simulink model "SEIRv2"  (R2019b)
settings: Solver=VariableStepAuto  StartTime=0.0  StopTime=365  FixedStep=1/24  RelTol=1e-6
settings Model: Creator=Alex  LastModifiedBy=Alex

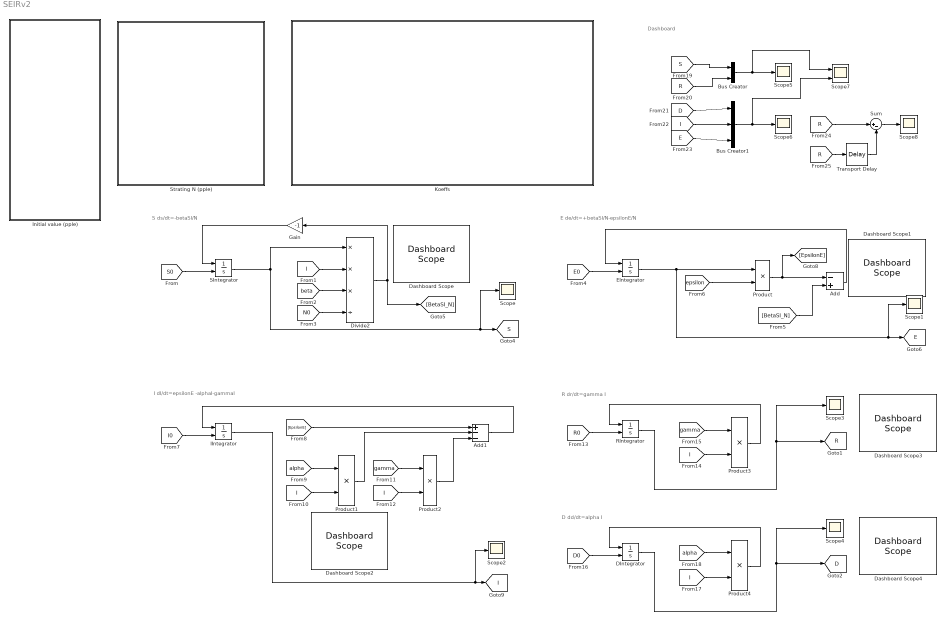
== system SEIRv2 ==
  note: Dashboard
  note: R dr/dt=gamma I
  note: I dI/dt=epsilonE -alphaI-gammaI
  note: E de/dt=+betaSI/N-epsilonE/N
  note: S ds/dt=-betaSI/N
  note: D dd/dt=alpha I
  Add : Sum  Inputs=-+
  Add1 : Sum  Inputs=+--
  Bus Creator : BusCreator  Inputs=2
  Bus Creator1 : BusCreator  Inputs=3
  DIntegrator : Integrator  InitialConditionSource=external
  Dashboard Scope{,1..4} (5 alike) : DashboardScope  Ymax=150e6
  Divide2 : Product  Inputs=***/
  EIntegrator : Integrator  InitialConditionSource=external
  Gain : Gain  Gain=-1
  IIntegrator : Integrator  InitialConditionSource=external
  Initial value (pple) : Subsystem
  Koeffs : Subsystem
  Product{,1..4} (5 alike) : Product  Inputs=**
  RIntegrator : Integrator  InitialConditionSource=external
  SIntegrator : Integrator  InitialConditionSource=external
  Scope{,1..6,8} (8 alike) : Scope
  Scope7 : Scope  NumInputPorts=2
  Strating N (pple) : Subsystem
  Sum : Sum  Inputs=|+-
  Transport Delay : TransportDelay
  tag scope: D=global, E=global, I=global, R=global, S=global
  wires:
  [S0] -> SIntegrator/2
  SIntegrator/1 -> Scope/1, [S], Divide2/1
  [I] -> Divide2/2
  [beta] -> Divide2/3
  [N0] -> Divide2/4
  Divide2/1 -> [BetaSI_N], Gain/1
  Gain/1 -> SIntegrator/1
  [E0] -> EIntegrator/2
  EIntegrator/1 -> Scope1/1, [E], Product/1
  [epsilon] -> Product/2
  Product/1 -> [EpsilonE], Add/1
  [BetaSI_N] -> Add/2
  Add/1 -> EIntegrator/1
  [I0] -> IIntegrator/2
  IIntegrator/1 -> [I], Scope2/1
  [alpha] -> Product1/1
  [I] -> Product1/2
  [gamma] -> Product2/1
  [I] -> Product2/2
  Product2/1 -> Add1/3
  Product1/1 -> Add1/2
  [EpsilonE] -> Add1/1
  Add1/1 -> IIntegrator/1
  [R0] -> RIntegrator/2
  RIntegrator/1 -> Scope3/1, [R]
  [gamma] -> Product3/1
  [I] -> Product3/2
  Product3/1 -> RIntegrator/1
  Product4/1 -> DIntegrator/1
  [I] -> Product4/2
  [alpha] -> Product4/1
  DIntegrator/1 -> [D], Scope4/1
  [D0] -> DIntegrator/2
  [S] -> Bus Creator/1
  [R] -> Bus Creator/2
  [D] -> Bus Creator1/1
  [I] -> Bus Creator1/2
  [E] -> Bus Creator1/3
  Bus Creator/1 -> Scope7/1, Scope5/1
  Bus Creator1/1 -> Scope7/2, Scope6/1
  [R] -> Transport Delay/1
  [R] -> Sum/1
  Transport Delay/1 -> Sum/2
  Sum/1 -> Scope8/1

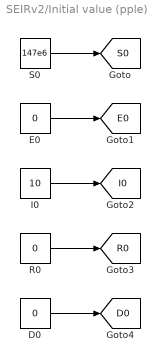
== system SEIRv2/Initial value (pple) ==
  D0 : Constant  Value=0
  E0 : Constant  Value=0
  I0 : Constant  Value=10
  R0 : Constant  Value=0
  S0 : Constant  Value=147e6
  tag scope: D0=global, E0=global, I0=global, R0=global, S0=global
  wires:
  S0/1 -> [S0]
  I0/1 -> [I0]
  D0/1 -> [D0]
  E0/1 -> [E0]
  R0/1 -> [R0]

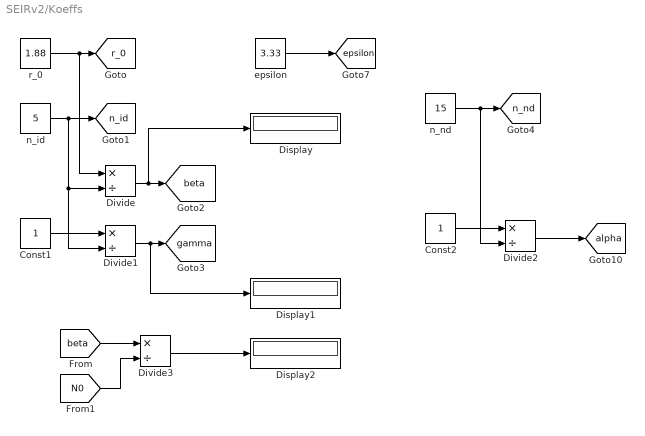
== system SEIRv2/Koeffs ==
  Const1 : Constant
  Const2 : Constant
  Display : Display
  Display1 : Display
  Display2 : Display
  Divide{,1..3} (4 alike) : Product  Inputs=*/
  epsilon : Constant  Value=3.33
  n_id : Constant  Value=5
  n_nd : Constant  Value=15
  r_0 : Constant  Value=1.88
  tag scope: alpha=global, beta=global, epsilon=global, gamma=global, n_id=global, n_nd=global, r_0=global
  wires:
  r_0/1 -> Divide/1, [r_0]
  Divide1/1 -> Display1/1, [gamma]
  n_id/1 -> Divide1/2, Divide/2, [n_id]
  Divide/1 -> Display/1, [beta]
  Const1/1 -> Divide1/1
  epsilon/1 -> [epsilon]
  Const2/1 -> Divide2/1
  Divide2/1 -> [alpha]
  n_nd/1 -> [n_nd], Divide2/2
  [beta] -> Divide3/1
  [N0] -> Divide3/2
  Divide3/1 -> Display2/1

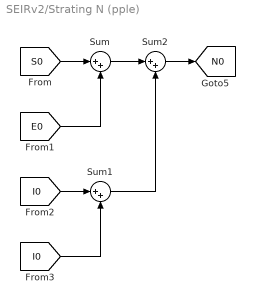
== system SEIRv2/Strating N (pple) ==
  Sum : Sum  Inputs=|++
  Sum1 : Sum  Inputs=|++
  Sum2 : Sum  Inputs=|++
  tag scope: N0=global
  wires:
  [I0] -> Sum1/1
  [S0] -> Sum/1
  [E0] -> Sum/2
  [I0] -> Sum1/2
  Sum2/1 -> [N0]
  Sum1/1 -> Sum2/2
  Sum/1 -> Sum2/1
